simulink model "RBF_neural_adaptive_controller_tele"  (R2023b)
settings: Solver=VariableStepAuto  StartTime=0.0  StopTime=20  RelTol=1e-3
settings Model: Creator=ASUS  LastModifiedBy=Arshia

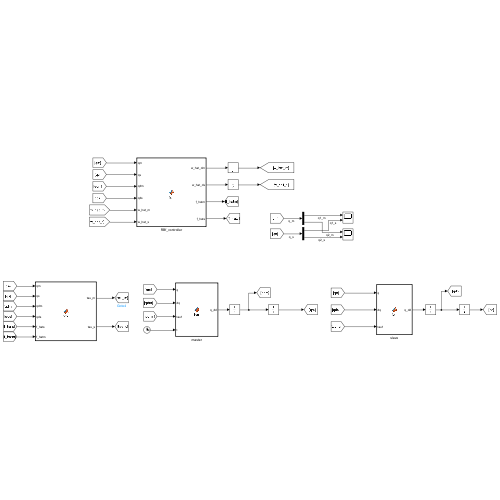
[thumbnail: Simulink's stored preview of the top-level diagram]
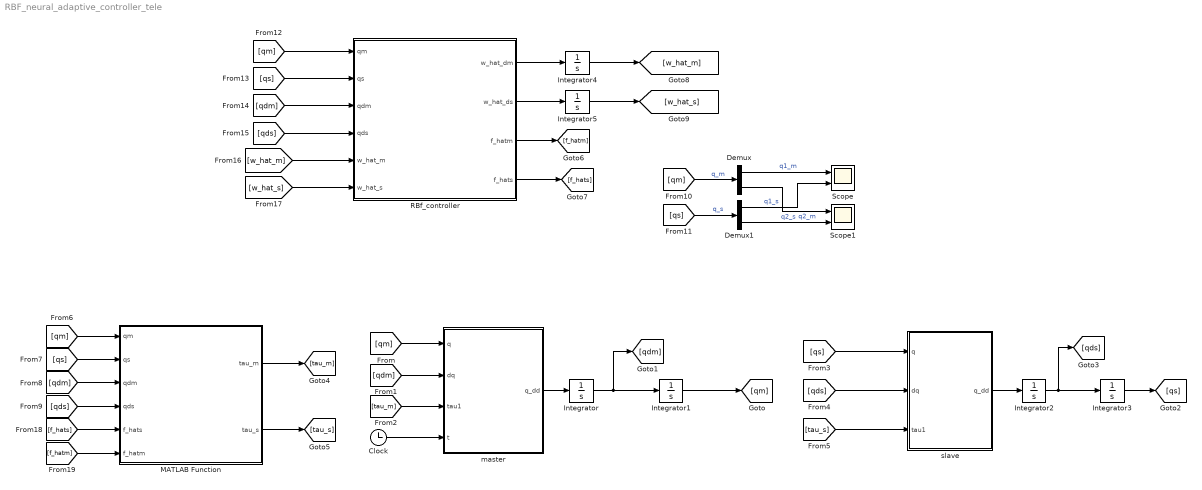
== system RBF_neural_adaptive_controller_tele ==
  Clock : Clock
  Demux : Demux  Outputs=2
  Demux1 : Demux  Outputs=2
  Integrator : Integrator  InitialCondition=zeros(2,1)
  Integrator1 : Integrator  InitialCondition=-[pi/4;pi/4]
  Integrator2 : Integrator  InitialCondition=zeros(2,1)
  Integrator3 : Integrator  InitialCondition=[pi/4;pi/4]
  Integrator4 : Integrator  InitialCondition=zeros(6,2)
  Integrator5 : Integrator  InitialCondition=zeros(6,2)
  MATLAB Function : MATLAB Function  TreatAsAtomicUnit=on
  RBf_controller : MATLAB Function  TreatAsAtomicUnit=on
  Scope : Scope  NumInputPorts=2
  Scope1 : Scope  NumInputPorts=2
  master : MATLAB Function  TreatAsAtomicUnit=on
  slave : MATLAB Function  TreatAsAtomicUnit=on
  wires:
  master/1(q_dd) -> Integrator/1
  Integrator/1 -> Integrator1/1, [qdm]
  Integrator1/1 -> [qm]
  [qm] -> master/1(q)
  [qdm] -> master/2(dq)
  [tau_m] -> master/3(tau1)
  slave/1(q_dd) -> Integrator2/1
  [qs] -> slave/1(q)
  Integrator3/1 -> [qs]
  Integrator2/1 -> Integrator3/1, [qds]
  [qds] -> slave/2(dq)
  [tau_s] -> slave/3(tau1)
  [qm] -> MATLAB Function/1(qm)
  [qs] -> MATLAB Function/2(qs)
  [qdm] -> MATLAB Function/3(qdm)
  [qds] -> MATLAB Function/4(qds)
  MATLAB Function/1(tau_m) -> [tau_m]
  MATLAB Function/2(tau_s) -> [tau_s]
  [qm] -> Demux/1  "q_m"
  Demux/1 -> Scope/1  "q1_m"
  Demux1/1 -> Scope/2  "q1_s"
  Demux/2 -> Scope1/1  "q2_m"
  Demux1/2 -> Scope1/2  "q2_s"
  [qs] -> Demux1/1  "q_s"
  Clock/1 -> master/4(t)
  RBf_controller/1(w_hat_dm) -> Integrator4/1
  RBf_controller/2(w_hat_ds) -> Integrator5/1
  RBf_controller/3(f_hatm) -> [f_hatm]
  RBf_controller/4(f_hats) -> [f_hats]
  Integrator4/1 -> [w_hat_m]
  Integrator5/1 -> [w_hat_s]
  [qm] -> RBf_controller/1(qm)
  [qs] -> RBf_controller/2(qs)
  [qdm] -> RBf_controller/3(qdm)
  [qds] -> RBf_controller/4(qds)
  [w_hat_m] -> RBf_controller/5(w_hat_m)
  [w_hat_s] -> RBf_controller/6(w_hat_s)
  [f_hats] -> MATLAB Function/5(f_hats)
  [f_hatm] -> MATLAB Function/6(f_hatm)

== matlab function RBF_neural_adaptive_controller_tele/slave ==
  data: q input; q_dd output; dq input; tau1 input
function q_dd = fcn(q,dq,tau1)

q1=q(1);
q2=q(2);

q1d=dq(1);
q2d=dq(2);



m1=.1;
m2=.1;

I1=.1;
I2=.1;

l1=.25;
l2=.12;

lc1=l1/2;
lc2=l2/2;


g=9.81;



d11=m1*lc1^2+m2*(l1^2+lc2^2+2*l1*lc2^2+2*l1*l2*cos(q2))+I1+I2;
d12=m2*(lc2^2+l1*l2*cos(q2))+I2;
d22=m2*lc2^2+I2;

h=-m2*l1*lc2*sin(q2);

c121=h;
c211=h;
c112=-h;
c221=h;



M=[d11,d12;d12,d22];
C=[c121*q2d,c211*q1d+c221*q2d;c112*q1d,0];
G=[(m1*lc1+m2*l1)*g*cos(q1)+m2*lc2*g*cos(q1+q2);m2*lc2*cos(q1+q2)];

    

 q_dd=pinv(M)*(-C*dq-G+tau1);

== matlab function RBF_neural_adaptive_controller_tele/master ==
  data: q input; q_dd output; dq input; tau1 input; t input
function q_dd = fcn(q,dq,tau1,t)

q1=q(1);
q2=q(2);

q1d=dq(1);
q2d=dq(2);



m1=.1;
m2=.1;

I1=.1;
I2=.1;

l1=.25;
l2=.12;

lc1=l1/2;
lc2=l2/2;


g=9.81;



d11=m1*lc1^2+m2*(l1^2+lc2^2+2*l1*lc2^2+2*l1*l2*cos(q2))+I1+I2;
d12=m2*(lc2^2+l1*l2*cos(q2))+I2;
d22=m2*lc2^2+I2;

h=-m2*l1*lc2*sin(q2);

c121=h;
c211=h;
c112=-h;
c221=h;



M=[d11,d12;d12,d22];
C=[c121*q2d,c211*q1d+c221*q2d;c112*q1d,0];
G=[(m1*lc1+m2*l1)*g*cos(q1)+m2*lc2*g*cos(q1+q2);m2*lc2*cos(q1+q2)];

%first input
% k=10;
%  q_des=sin(t)*ones(2,1);
%  qd_des=cos(t)*ones(2,1);
%  tauh1=-k*(q-q_des)-k*(dq-qd_des);

 %second input
 k=10;
 if t>=0 && t<5
 q_des=[pi/2;pi];
 qd_des=zeros(2,1);
 tauh1=-k*(q-q_des)-k*(dq-qd_des);

 elseif t>=5 && t<10
 q_des=[-pi/2;-pi];
 qd_des=zeros(2,1);
 tauh1=-k*(q-q_des)-k*(dq-qd_des);
 else

 q_des=[0;pi/8];
 qd_des=zeros(2,1);
 tauh1=-k*(q-q_des)-k*(dq-qd_des);
 end


 
 q_dd=pinv(M)*(-C*dq-G+tau1+tauh1);

== matlab function RBF_neural_adaptive_controller_tele/MATLAB Function ==
  data: qm input; tau_m output; qs input; qdm input; qds input; tau_s output; f_hats input; f_hatm input
function [tau_m,tau_s] = fcn(qm,qs,qdm,qds,f_hats,f_hatm)
landa=30;
em=qm-qs;
edm=qdm-qds;
rm=edm+landa*em;

es=qs-qm;
eds=qds-qdm;
rs=eds+landa*es;

Km=5*eye(2);
tau_m=-Km*rm+f_hatm;


Ks=5*eye(2);
tau_s=-Ks*rs+f_hats;

== matlab function RBF_neural_adaptive_controller_tele/RBf_controller ==
  data: qm input; w_hat_dm output; qs input; qdm input; qds input; w_hat_m input; w_hat_s input; w_hat_ds output; f_hatm output; f_hats output
function  [w_hat_dm,w_hat_ds,f_hatm,f_hats]= fcn(qm,qs,qdm,qds,w_hat_m,w_hat_s)







%master
landa=30;
em=qm-qs;
edm=qdm-qds;
rm=edm+landa*em;
x=[qm;qdm];
mu1=.1*ones(4,1);
sigma1=2;
phi1=exp(-norm(x-mu1)^2/(sigma1));
p=3;
Phi1=phi1*ones(p,1);

mu2=.5*ones(4,1);
sigma2=3;
phi2=exp(-norm(x-mu2)^2/(sigma2));
p=3;
Phi2=phi2*ones(p,1);

Phi=[Phi1;Phi2];

n=2;
Qm=10*eye(n*p);
Bm=5*eye(n*p);

w_hat_dm=-(pinv(Qm))'*Phi*rm'-(pinv(Qm))'*Bm*w_hat_m;
f_hatm=w_hat_m'*Phi;

%slave
es=qs-qm;
eds=qds-qdm;
rs=eds+landa*es;
x=[qs;qs];
mu1=.1*ones(4,1);
sigma1=2;
phi1=exp(-norm(x-mu1)^2/(sigma1));
p=3;
Phi1=phi1*ones(p,1);

mu2=.5*ones(4,1);
sigma2=3;
phi2=exp(-norm(x-mu2)^2/(sigma2));
p=3;
Phi2=phi2*ones(p,1);

Phi=[Phi1;Phi2];

n=2;
Qs=10*eye(n*p);
Bs=5*eye(n*p);

w_hat_ds=-(pinv(Qs))'*Phi*rs'-(pinv(Qm))'*Bs*w_hat_s;
f_hats=w_hat_s'*Phi;
